simulink model "Wind_power_plant_model"  (R2020a)
settings: Solver=FixedStepAuto  StartTime=0.0  StopTime=30.0  FixedStep=0.001  RelTol=1e-3
libraries: powerlib x7, re_lib x1
settings Model: Creator=Reaga  LastModifiedBy=Reaga
settings DebuggingCC: UnconnectedInputMsg=none  UnconnectedOutputMsg=none  UnconnectedLineMsg=none
settings ModelReferenceCC: EnableRefExpFcnMdlSchedulingChecks=off
settings RTWCC: Description=Generic Real-Time Target
settings ConfigComp: CovBoundaryAbsTol=1.0e-5

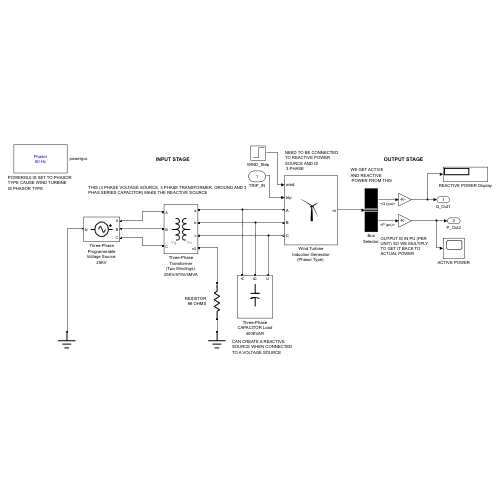
[thumbnail: Simulink's stored preview of the top-level diagram]
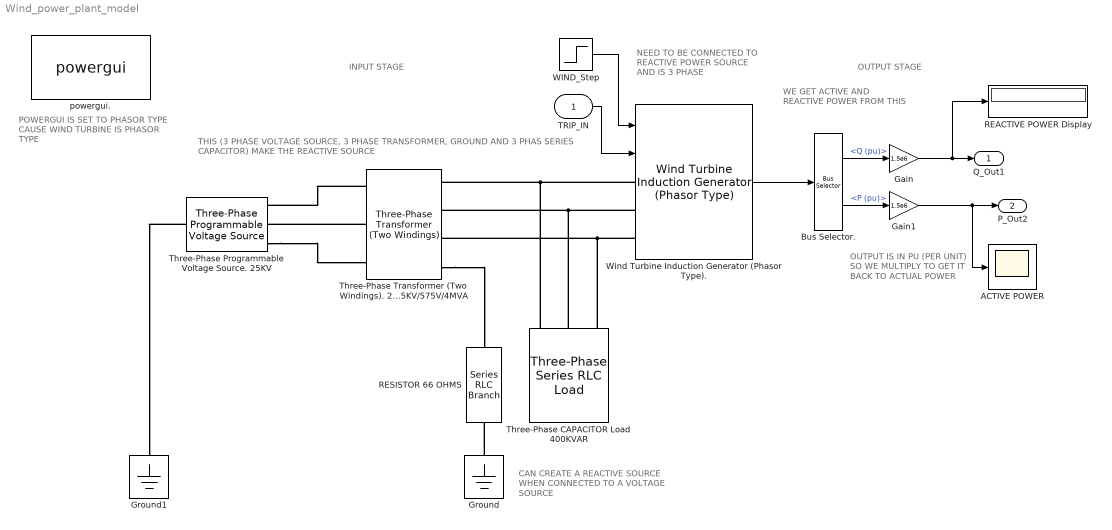
== system Wind_power_plant_model ==
  note: POWERGUI IS SET TO PHASOR
      | TYPE CAUSE WIND TURBINE
      | IS PHASOR TYPE
  note: OUTPUT IS IN PU (PER UNIT) SO WE MULTIPLY TO GET IT BACK TO ACTUAL POWER
  note: WE GET ACTIVE
      | AND REACTIVE
      |  POWER FROM THIS
  note: INPUT STAGE
  note: OUTPUT STAGE
  note: THIS (3 PHASE VOLTAGE SOURCE, 3 PHASE TRANSFORMER, GROUND AND 3 PHAS SERIES CAPACITOR) MAKE THE REACTIVE SOURCE
  note: CAN CREATE A REACTIVE
      | SOURCE WHEN CONNECTED
      | TO A VOLTAGE SOURCE
  note: NEED TO BE CONNECTED
      | TO REACTIVE POWER
      | SOURCE AND IS
      |  3 PHASE
  TRIP_IN : Inport
  ACTIVE POWER : Scope
  Bus Selector. : BusSelector  OutputSignals=Q (pu),P (pu)
  Gain : Gain  Gain=1.5e6
  Gain1 : Gain  Gain=1.5e6
  Ground : powerlib/Elements/Ground  LConnTagsString=a
  Ground1 : powerlib/Elements/Ground  LConnTagsString=a
  REACTIVE POWER Display : Display
  RESISTOR 66 OHMS : powerlib/Elements/Series RLC Branch  LConnTagsString=__new0  RConnTagsString=__new0  BranchType=R  Resistance=66  Inductance=1e-3  SetiL0=off  InitialCurrent=0  Capacitance=1e-6  Setx0=off  InitialVoltage=0  Measurements=None
  Three-Phase CAPACITOR Load 400KVAR : powerlib/Elements/Three-Phase Series RLC Load  LConnTagsString=A|B|C  Configuration=Delta  NominalVoltage=575  Vabc=[1e3 1e3 1e3]  Vabcp=[1e3 1e3 1e3]  NominalFrequency=60  UnbalancedPower=off  ActivePower=0  InductivePower=0  CapacitivePower=400e3  Pabc=[10e3 9e3 11e3]  QLabc=[100 90 110]  QCabc=[100 90 110]  Pabcp=[10e3 9e3 11e3]  QLabcp=[100 90 110]  QCabcp=[100 90 110]  Measurements=None  LoadType=constant Z
  Three-Phase Programmable Voltage Source. 25KV : powerlib/Electrical Sources/Three-Phase Programmable Voltage Source  PositiveSequence="[25e3  0 60]"  VariationEntity=None  VariationType=Table of time-amplitude pairs  VariationTypeAlt=Step  VariationStep=0.5  VariationRate=10  VariationMagnitude=0.3  VariationFrequency=2  VariationTiming=[1 2]  VariationPhaseA=off  Amplitudes=[1 0.8 1.2 1.0]  TimeValues=[0 0.1 0.15 0.2]  HarmonicGeneration=off  HarmonicA=[3 0.2 -25 0]  HarmonicB=[2 0.15 35 2]  Timing="[0.05  3]"  BusType=swing  Pref=0  Qref=0  Qmin=-inf  Qmax=inf
  Three-Phase Transformer (Two Windings). 25KV/575V/4MVA : powerlib/Elements/Three-Phase Transformer (Two Windings)  Winding1Connection=Yg  Winding2Connection=Yn  CoreType=Three single-phase transformers  SetSaturation=off  Hysteresis=off  DataFile='hysteresis'  SetInitialFlux=off  Measurements=None  UNITS=pu  NominalPower=[ 4e6 , 60 ]  Winding1=[ 25e3 , 0.025/30 , 0.025 ]  Winding2=[ 575 , 0.025/30 , 0.025 ]  Rm=500  Lm=Inf  L0=0.5  Saturation=[ 0,0 ; 0.0024,1.2 ; 1.0,1.52 ]  InitialFluxes=[ 0.8 , -0.8 , 0.7 ]  BreakLoop=off  DiscreteSolver=Trapezoidal iterative  DataType=off  TransfoNumber=1
  WIND_Step : Step  After=12  SampleTime=0
  Wind Turbine Induction Generator (Phasor Type). : re_lib/Wind Generation/Wind Turbine Induction Generator (Phasor Type)  ExternalTm=off  nom=[1.5e6, 575, 60]  sta=[ 0.004843, 0.1248]  rot=[ 0.004377, 0.1791]  Lm=6.77  mec=[5.04, 0.01, 3]  init="[ -0.01,0,   0,0,0,   0,0,0 ]"  pitch_angle=0  Pmec=1.5e6  wind_base=12  speed_nom=1  P_wind_base=1  K_pitch_gain=[5 25]  pitch_max=45  pitch_rate=2
  powergui. : powerlib/powergui  Priority=1  SimulationMode=Phasor  SampleTime=50e-6  frequency=60  Iterations=50  frequencyindice=60  Pbase=10e6  ErrMax=1e-4  UnitsV=V  UnitsW=W  buscounter=0  FunctionMessages=off  echomessages=off  EnableUseOfTLC=off  CurrentSourceSwitches=off  DisableSnubberDevices=off  DisableRonSwitches=off  DisableVfSwitches=off  DisplayEquations=off  AutomaticDiscreteSolvers=off  SolverType=Tustin/Backward Euler (TBE)  Interpol=off  ExternalGateDelay=off  methode=off  Ts=100  x0status=blocks  SPID=on  SwTol=0  HookPort=off  NonlinearTolerance=1e-4  nMaxIteration=100  ContinueOnMaxIteration=off  RestoreLinks=warning  ResistiveCurrentMeasurement=off  Frange=[0:2:500]  Ylog=off  Xlog=on  ShowGrid=off  save=off  variable=ZData  structure=0  ZoomFFT=off  StartTime=0.0  cycles=1  DisplayStyle=1  fundamental=60  FreqAxis=off  MaxFrequency=1000  frequencyindicesteady=1  RmsSteady=1  display=off
  Q_Out1 : Outport
  P_Out2 : Outport  Port=2
  wires:
  Wind Turbine Induction Generator (Phasor Type)./1 -> Bus Selector./1
  Bus Selector./1 -> Gain/1  "<Q (pu)>"
  Bus Selector./2 -> Gain1/1  "<P (pu)>"
  Gain/1 -> REACTIVE POWER Display/1, Q_Out1/1
  Gain1/1 -> ACTIVE POWER/1, P_Out2/1
  TRIP_IN/1 -> Wind Turbine Induction Generator (Phasor Type)./2
  WIND_Step/1 -> Wind Turbine Induction Generator (Phasor Type)./1
  connections:
  Three-Phase Transformer (Two Windings). 25KV/575V/4MVA/RConn4 -- RESISTOR 66 OHMS/LConn1
  Ground/LConn1 -- RESISTOR 66 OHMS/RConn1
  Three-Phase Programmable Voltage Source. 25KV/LConn1 -- Ground1/LConn1
  Three-Phase Transformer (Two Windings). 25KV/575V/4MVA/LConn1 -- Three-Phase Programmable Voltage Source. 25KV/RConn1
  Three-Phase Transformer (Two Windings). 25KV/575V/4MVA/LConn2 -- Three-Phase Programmable Voltage Source. 25KV/RConn2
  Three-Phase Programmable Voltage Source. 25KV/RConn3 -- Three-Phase Transformer (Two Windings). 25KV/575V/4MVA/LConn3
  Wind Turbine Induction Generator (Phasor Type)./LConn3 -- Three-Phase CAPACITOR Load 400KVAR/LConn3 -- Three-Phase Transformer (Two Windings). 25KV/575V/4MVA/RConn3
  Wind Turbine Induction Generator (Phasor Type)./LConn2 -- Three-Phase CAPACITOR Load 400KVAR/LConn2 -- Three-Phase Transformer (Two Windings). 25KV/575V/4MVA/RConn2
  Wind Turbine Induction Generator (Phasor Type)./LConn1 -- Three-Phase CAPACITOR Load 400KVAR/LConn1 -- Three-Phase Transformer (Two Windings). 25KV/575V/4MVA/RConn1
